simulink library "csc_spc_sensor_processing_lib"  (R2014b)
settings: Solver=ode45  StartTime=0.0  StopTime=10.0  RelTol=1e-3
undefined symbols (not defined in the file): kfl_use_mems, mnm_accel_range, mnm_gyro_range
libraries: util_info_lib x1
settings Model: Creator=escrane  LastModifiedBy=mstewart

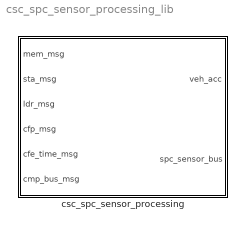
== system csc_spc_sensor_processing_lib ==
  csc_spc_sensor_processing : Subsystem

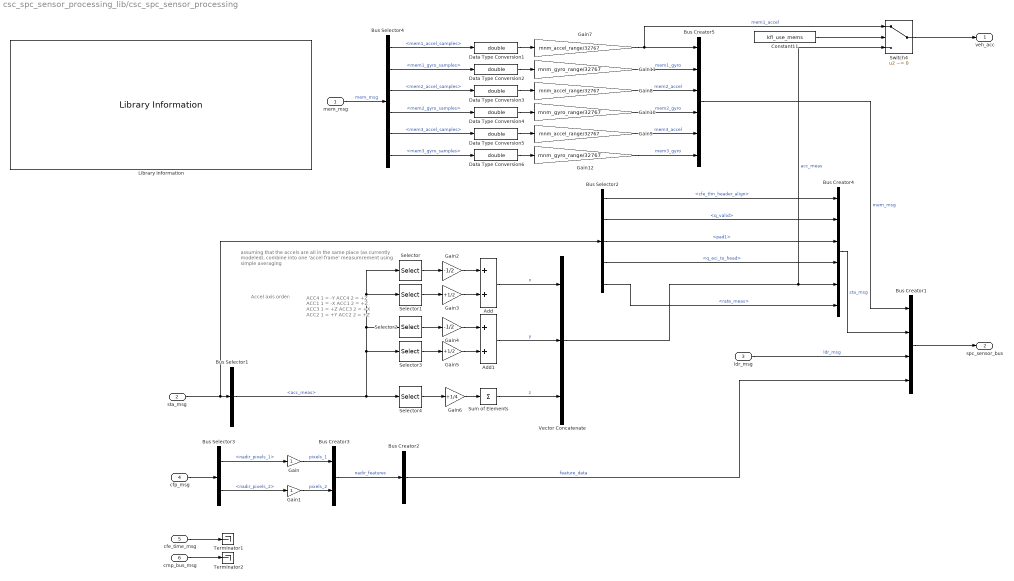
== system csc_spc_sensor_processing_lib/csc_spc_sensor_processing ==
  note: ACC4 1 = -Y
      | ACC4 2 = +Z
      | ACC1 1 = -X
      | ACC1 2 = +Z
      | ACC3 1 = +Z
      | ACC3 2 = +X
      | ACC2 1 = +Y
      | ACC2 2 = +Z
  note: assuming that the accels are all in the same place
      | (as currently modeled), combine into one 'accel frame'
      | measumrement using simple averaging
  note: Accel axis order:
  mem_msg : Inport
  sta_msg : Inport  Port=2
  ldr_msg : Inport  Port=3
  cfp_msg : Inport  Port=4
  cfe_time_msg : Inport  Port=5
  cmp_bus_msg : Inport  Port=6
  Add : Sum
  Add1 : Sum
  Bus Creator1 : BusCreator
  Bus Creator2 : BusCreator  Inputs=1
  Bus Creator3 : BusCreator  Inputs=2
  Bus Creator4 : BusCreator  Inputs=6
  Bus Creator5 : BusCreator  Inputs=6
  Bus Selector1 : BusSelector  OutputSignals=acc_meas
  Bus Selector2 : BusSelector  OutputSignals=cfe_tlm_header_align,q_valid,pad1,q_eci_to_head,rate_meas
  Bus Selector3 : BusSelector  OutputSignals=nadir_pixels_1,nadir_pixels_2
  Bus Selector4 : BusSelector  OutputSignals=mem1_accel_samples,mem1_gyro_samples,mem2_accel_samples,mem2_gyro_samples,mem3_accel_samples,mem3_gyro_samples
  Constant11 : Constant  Value=kfl_use_mems
  Data Type Conversion{1..6} (6 alike) : DataTypeConversion  OutDataTypeStr=double
  Gain : Gain
  Gain1 : Gain
  Gain10 : Gain  Gain=mnm_gyro_range/32767
  Gain11 : Gain  Gain=mnm_gyro_range/32767
  Gain12 : Gain  Gain=mnm_gyro_range/32767
  Gain2 : Gain  Gain=-1/2
  Gain3 : Gain  Gain=+1/2
  Gain4 : Gain  Gain=-1/2
  Gain5 : Gain  Gain=+1/2
  Gain6 : Gain  Gain=+1/4
  Gain7 : Gain  Gain=mnm_accel_range/32767
  Gain8 : Gain  Gain=mnm_accel_range/32767
  Gain9 : Gain  Gain=mnm_accel_range/32767
  Library Information : util_info_lib/Library Information  owner='escrane'
  Selector : Selector  NumberOfDimensions=2  InputPortWidth=3  IndexOptions=Select all,Index vector (dialog)  Indices=[3],[ 3 ]  OutputSizes=1,1
  Selector1 : Selector  NumberOfDimensions=2  InputPortWidth=3  IndexOptions=Select all,Index vector (dialog)  Indices=[6],[6]  OutputSizes=1,1
  Selector2 : Selector  NumberOfDimensions=2  InputPortWidth=3  IndexOptions=Select all,Index vector (dialog)  Indices=[1],[1]  OutputSizes=1,1
  Selector3 : Selector  NumberOfDimensions=2  InputPortWidth=3  IndexOptions=Select all,Index vector (dialog)  Indices=[7],[7]  OutputSizes=1,1
  Selector4 : Selector  NumberOfDimensions=2  InputPortWidth=3  IndexOptions=Select all,Index vector (dialog)  Indices=[2 4 5 8],[2 4 5 8]  OutputSizes=1,1
  Sum of Elements : Sum  Inputs=+  CollapseMode=Specified dimension  CollapseDim=2
  Switch4 : Switch  Criteria=u2 ~= 0
  Terminator1 : Terminator
  Terminator2 : Terminator
  Vector Concatenate : Concatenate  NumInputs=3  Mode=Multidimensional array  ConcatenateDimension=2
  veh_acc : Outport
  spc_sensor_bus : Outport  Port=2
  wires:
  Switch4/1 -> veh_acc/1
  Constant11/1 -> Switch4/2
  Gain9/1 -> Bus Creator5/5  "mem3_accel"
  Gain12/1 -> Bus Creator5/6  "mem3_gyro"
  Gain10/1 -> Bus Creator5/4  "mem2_gyro"
  Gain8/1 -> Bus Creator5/3  "mem2_accel"
  Gain11/1 -> Bus Creator5/2  "mem1_gyro"
  Gain7/1 -> Bus Creator5/1, Switch4/1  "mem1_accel"
  Data Type Conversion6/1 -> Gain12/1
  Data Type Conversion5/1 -> Gain9/1
  Data Type Conversion4/1 -> Gain10/1
  Data Type Conversion3/1 -> Gain8/1
  Data Type Conversion2/1 -> Gain11/1
  Data Type Conversion1/1 -> Gain7/1
  Bus Selector4/6 -> Data Type Conversion6/1  "<mem3_gyro_samples>"
  Bus Selector4/5 -> Data Type Conversion5/1  "<mem3_accel_samples>"
  Bus Selector4/4 -> Data Type Conversion4/1  "<mem2_gyro_samples>"
  Bus Selector4/3 -> Data Type Conversion3/1  "<mem2_accel_samples>"
  Bus Selector4/2 -> Data Type Conversion2/1  "<mem1_gyro_samples>"
  Bus Selector4/1 -> Data Type Conversion1/1  "<mem1_accel_samples>"
  mem_msg/1 -> Bus Selector4/1  "mem_msg"
  Bus Creator5/1 -> Bus Creator1/1  "mem_msg"
  Vector Concatenate/1 -> Bus Creator4/5, Switch4/3  "acc_meas"
  Bus Selector2/5 -> Bus Creator4/6  "<rate_meas>"
  Bus Selector2/4 -> Bus Creator4/4  "<q_eci_to_head>"
  Bus Selector2/3 -> Bus Creator4/3  "<pad1>"
  Bus Selector2/2 -> Bus Creator4/2  "<q_valid>"
  Bus Selector2/1 -> Bus Creator4/1  "<cfe_tlm_header_align>"
  Bus Creator4/1 -> Bus Creator1/2  "sta_msg"
  Sum of Elements/1 -> Vector Concatenate/3  "z"
  Gain6/1 -> Sum of Elements/1
  Selector4/1 -> Gain6/1
  Add1/1 -> Vector Concatenate/2  "y"
  Gain5/1 -> Add1/2
  Gain4/1 -> Add1/1
  Selector3/1 -> Gain5/1
  Selector2/1 -> Gain4/1
  Add/1 -> Vector Concatenate/1  "x"
  Gain3/1 -> Add/2
  Gain2/1 -> Add/1
  Selector1/1 -> Gain3/1
  Selector/1 -> Gain2/1
  Bus Selector1/1 -> Selector3/1, Selector/1, Selector1/1, Selector2/1, Selector4/1  "<acc_meas>"
  sta_msg/1 -> Bus Selector1/1, Bus Selector2/1
  ldr_msg/1 -> Bus Creator1/3  "ldr_msg"
  cfp_msg/1 -> Bus Selector3/1
  Bus Creator2/1 -> Bus Creator1/4  "feature_data"
  Bus Selector3/2 -> Gain1/1  "<nadir_pixels_2>"
  Bus Selector3/1 -> Gain/1  "<nadir_pixels_1>"
  Gain/1 -> Bus Creator3/1  "pixels_1"
  Gain1/1 -> Bus Creator3/2  "pixels_2"
  Bus Creator3/1 -> Bus Creator2/1  "nadir_features"
  cfe_time_msg/1 -> Terminator1/1
  cmp_bus_msg/1 -> Terminator2/1
  Bus Creator1/1 -> spc_sensor_bus/1
